simulink model "boot_model"  (R2018b)
settings: Solver=VariableStepAuto  StartTime=0.0  StopTime=0.02  RelTol=1e-3
undefined symbols (not defined in the file or in its folder): C, L, R
libraries: simulink x2, powerlib_meascontrol x2
settings Model: Creator=zjc81  LastModifiedBy=zjc81

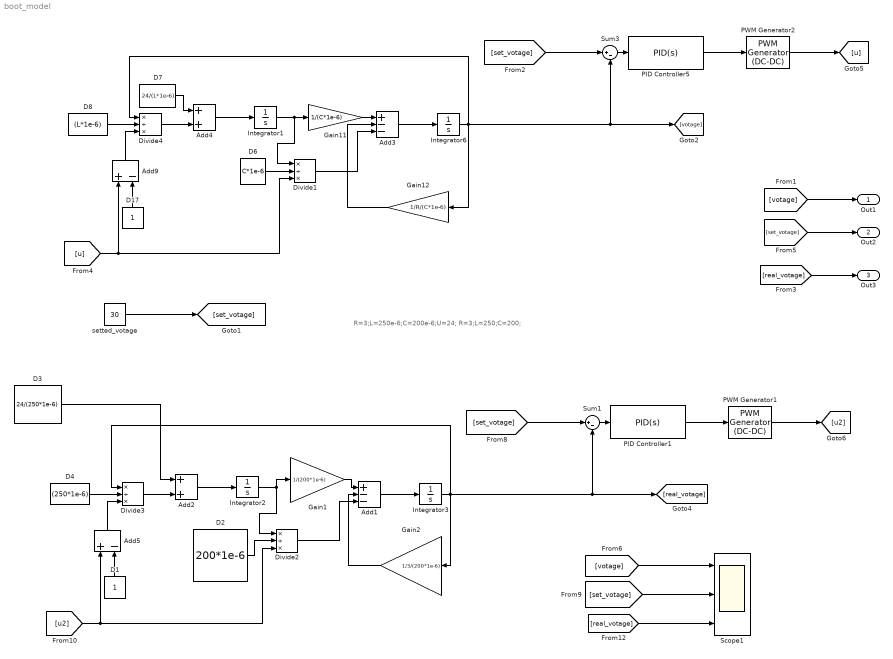
== system boot_model ==
  note: R=3;L=250e-6;C=200e-6;U=24;
      | R=3;L=250;C=200;
  Add1 : Sum  Inputs=+--
  Add2 : Sum
  Add3 : Sum  Inputs=+--
  Add4 : Sum
  Add5 : Sum  Inputs=+-
  Add9 : Sum  Inputs=+-
  D1 : Constant
  D17 : Constant
  D2 : Constant  Value=200*1e-6
  D3 : Constant  Value=24/(250*1e-6)
  D4 : Constant  Value=(250*1e-6)
  D6 : Constant  Value=C*1e-6
  D7 : Constant  Value=24/(L*1e-6)
  D8 : Constant  Value=(L*1e-6)
  Divide{1..4} (4 alike) : Product  Inputs=*/*
  Gain1 : Gain  Gain=1/(200*1e-6)
  Gain11 : Gain  Gain=1/(C*1e-6)
  Gain12 : Gain  Gain=1/R/(C*1e-6)
  Gain2 : Gain  Gain=1/3/(200*1e-6)
  Integrator{1..3,6} (4 alike) : Integrator
  PID Controller1 : simulink/Continuous/PID Controller  Controller=PID  Form=Parallel  TimeDomain=Continuous-time  SampleTime=-1  IntegratorMethod=Forward Euler  FilterMethod=Forward Euler  ControllerParametersSource=internal  P=0.0036  I=7.5  D=0  UseFilter=on  N=100  TunerSelectOption=Transfer Function Based (PID Tuner App)  InitialConditionSource=internal  InitialConditionForIntegrator=0  InitialConditionForFilter=0  DifferentiatorICPrevScaledInput=0  ExternalReset=none  TrackingMode=off  Kt=1  LimitOutput=on  UpperSaturationLimit=0.98  LowerSaturationLimit=0.02  LinearizeAsGain=on  AntiWindupMode=none  Kb=1  POutMin=[]  POutMax=[]  IOutMin=[]  IOutMax=[]  DOutMin=[]  DOutMax=[]  NOutMin=[]  NOutMax=[]  SumOutMin=[]  SumOutMax=[]  SaturationOutMin=[]  SaturationOutMax=[]  PParamMin=[]  PParamMax=[]  IParamMin=[]  IParamMax=[]  DParamMin=[]  DParamMax=[]  NParamMin=[]  NParamMax=[]  KbParamMin=[]  KbParamMax=[]  KtParamMin=[]  KtParamMax=[]  KbOutMin=[]  KbOutMax=[]  KtOutMin=[]  KtOutMax=[]  IntegratorOutMin=[]  IntegratorOutMax=[]  FilterOutMin=[]  FilterOutMax=[]  SumI1OutMin=[]  SumI1OutMax=[]  SumI2OutMin=[]  SumI2OutMax=[]  SumI3OutMin=[]  SumI3OutMax=[]  SumI4OutMin=[]  SumI4OutMax=[]  SumDOutMin=[]  SumDOutMax=[]  DifferentiatorOutMin=[]  DifferentiatorOutMax=[]  FilterDiffOutCoefMin=[]  FilterDiffOutCoefMax=[]  ReciprocalOutMin=[]  ReciprocalOutMax=[]  SumDenOutMin=[]  SumDenOutMax=[]  SumNumOutMin=[]  SumNumOutMax=[]  DivideOutMin=[]  DivideOutMax=[]  IntegratorContinuousStateAttributes=''  IntegratorStateMustResolveToSignalObject=off  IntegratorRTWStateStorageClass=Auto  FilterContinuousStateAttributes=''  FilterStateMustResolveToSignalObject=off  FilterRTWStateStorageClass=Auto  ParallelPVariant=InternalParameters  IdealPVariant=Disabled  IVariant=InternalParameters  DVariant=InternalParameters  IntegratorVariant=Continuous  SatVariant=Enabled  AWVariant=Passthrough  PCopyVariant=Disabled  TRVariant=Disabled  FdbkBlocksVariant=Forward  IdealPFdbkVariant=Disabled  SatFdbkVariant=Disabled  DerivativeFilterVariant=ContFilter  NVariant=InternalParameters  NCopyVariant=Disabled  FilterICVariant=InternalICsFilter  IntegratorICVariant=InternalICs  ExternalResetVariant=Disabled  TRSumVariant=Passthrough  SumFdbkVariant=Disabled  SumVariant=Sum_PID
  PID Controller5 : simulink/Continuous/PID Controller  Controller=PID  Form=Parallel  TimeDomain=Continuous-time  SampleTime=-1  IntegratorMethod=Forward Euler  FilterMethod=Forward Euler  ControllerParametersSource=internal  P=0.0036  I=7.5  D=0  UseFilter=on  N=100  TunerSelectOption=Transfer Function Based (PID Tuner App)  InitialConditionSource=internal  InitialConditionForIntegrator=0  InitialConditionForFilter=0  DifferentiatorICPrevScaledInput=0  ExternalReset=none  TrackingMode=off  Kt=1  LimitOutput=on  UpperSaturationLimit=0.98  LowerSaturationLimit=0.02  LinearizeAsGain=on  AntiWindupMode=none  Kb=1  POutMin=[]  POutMax=[]  IOutMin=[]  IOutMax=[]  DOutMin=[]  DOutMax=[]  NOutMin=[]  NOutMax=[]  SumOutMin=[]  SumOutMax=[]  SaturationOutMin=[]  SaturationOutMax=[]  PParamMin=[]  PParamMax=[]  IParamMin=[]  IParamMax=[]  DParamMin=[]  DParamMax=[]  NParamMin=[]  NParamMax=[]  KbParamMin=[]  KbParamMax=[]  KtParamMin=[]  KtParamMax=[]  KbOutMin=[]  KbOutMax=[]  KtOutMin=[]  KtOutMax=[]  IntegratorOutMin=[]  IntegratorOutMax=[]  FilterOutMin=[]  FilterOutMax=[]  SumI1OutMin=[]  SumI1OutMax=[]  SumI2OutMin=[]  SumI2OutMax=[]  SumI3OutMin=[]  SumI3OutMax=[]  SumI4OutMin=[]  SumI4OutMax=[]  SumDOutMin=[]  SumDOutMax=[]  DifferentiatorOutMin=[]  DifferentiatorOutMax=[]  FilterDiffOutCoefMin=[]  FilterDiffOutCoefMax=[]  ReciprocalOutMin=[]  ReciprocalOutMax=[]  SumDenOutMin=[]  SumDenOutMax=[]  SumNumOutMin=[]  SumNumOutMax=[]  DivideOutMin=[]  DivideOutMax=[]  IntegratorContinuousStateAttributes=''  IntegratorStateMustResolveToSignalObject=off  IntegratorRTWStateStorageClass=Auto  FilterContinuousStateAttributes=''  FilterStateMustResolveToSignalObject=off  FilterRTWStateStorageClass=Auto  ParallelPVariant=InternalParameters  IdealPVariant=Disabled  IVariant=InternalParameters  DVariant=InternalParameters  IntegratorVariant=Continuous  SatVariant=Enabled  AWVariant=Passthrough  PCopyVariant=Disabled  TRVariant=Disabled  FdbkBlocksVariant=Forward  IdealPFdbkVariant=Disabled  SatFdbkVariant=Disabled  DerivativeFilterVariant=ContFilter  NVariant=InternalParameters  NCopyVariant=Disabled  FilterICVariant=InternalICsFilter  IntegratorICVariant=InternalICs  ExternalResetVariant=Disabled  TRSumVariant=Passthrough  SumFdbkVariant=Disabled  SumVariant=Sum_PID
  PWM Generator1 : powerlib_meascontrol/Pulse & Signal Generators/PWM Generator (DC-DC)  Fsw=20e3  Ts=0
  PWM Generator2 : powerlib_meascontrol/Pulse & Signal Generators/PWM Generator (DC-DC)  Fsw=20e3  Ts=0
  Scope1 : Scope  NumInputPorts=3
  Sum1 : Sum  Inputs=|+-
  Sum3 : Sum  Inputs=|+-
  setted_votage : Constant  Value=30
  Out1 : Outport  SampleTime=1e-6
  Out2 : Outport  Port=2  SampleTime=1e-6
  Out3 : Outport  Port=3  SampleTime=1e-6
  wires:
  D7/1 -> Add4/1
  setted_votage/1 -> [set_votage]
  D6/1 -> Divide1/2
  [set_votage] -> Sum3/1
  Integrator1/1 -> Divide1/1, Gain11/1
  Gain11/1 -> Add3/1
  Add3/1 -> Integrator6/1
  Divide1/1 -> Add3/3
  PWM Generator2/1 -> [u]
  PID Controller5/1 -> PWM Generator2/1
  [u] -> Divide1/3, Add9/1
  Add4/1 -> Integrator1/1
  Divide4/1 -> Add4/2
  D8/1 -> Divide4/2
  D17/1 -> Add9/2
  Sum3/1 -> PID Controller5/1
  Add9/1 -> Divide4/3
  Integrator6/1 -> [votage], Sum3/2, Divide4/1, Gain12/1
  Gain12/1 -> Add3/2
  [votage] -> Out1/1
  [set_votage] -> Out2/1
  [votage] -> Scope1/1
  Gain2/1 -> Add1/2
  Integrator3/1 -> Gain2/1, Divide3/1, Sum1/2, [real_votage]
  Add5/1 -> Divide3/3
  Sum1/1 -> PID Controller1/1
  D1/1 -> Add5/2
  D4/1 -> Divide3/2
  Divide3/1 -> Add2/2
  Add2/1 -> Integrator2/1
  [u2] -> Add5/1, Divide2/3
  PID Controller1/1 -> PWM Generator1/1
  PWM Generator1/1 -> [u2]
  Divide2/1 -> Add1/3
  Add1/1 -> Integrator3/1
  Gain1/1 -> Add1/1
  Integrator2/1 -> Gain1/1, Divide2/1
  [set_votage] -> Sum1/1
  D2/1 -> Divide2/2
  D3/1 -> Add2/1
  [set_votage] -> Scope1/2
  [real_votage] -> Scope1/3
  [real_votage] -> Out3/1
